simulink model "A_CT_ur10"  (R2021b)
settings: Solver=FixedStepAuto  StartTime=0.0  StopTime=15  FixedStep=1e-3  RelTol=1e1
values from neighbouring files (symbols this model uses):
  Kp = 28*diag([14 14 17 10 22 22])    [GuadagniControllore.m]
  Kv = 32*diag([14 14 17 10 22 22])    [GuadagniControllore.m]
undefined symbols (not defined in the file or in its folder): l1, l2, l3, l4, l5, l6, m1, m2, m3, m4, m5, m6, q0, r
libraries: roblocks x3
(part 1 of 5)
settings Model: Creator=pierg  LastModifiedBy=pierg
settings ModelReferenceCC: ModelReferenceMinAlgLoopOccurrences=on

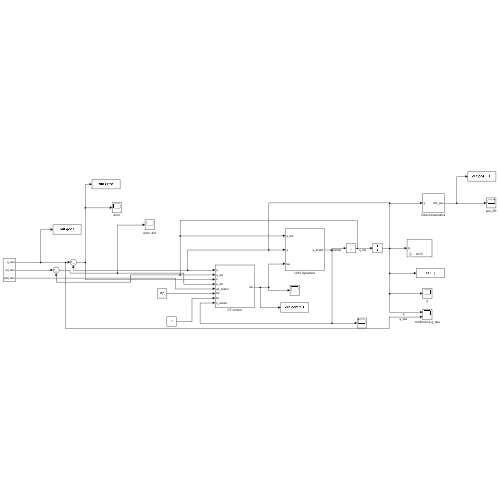
[thumbnail: Simulink's stored preview of the top-level diagram]
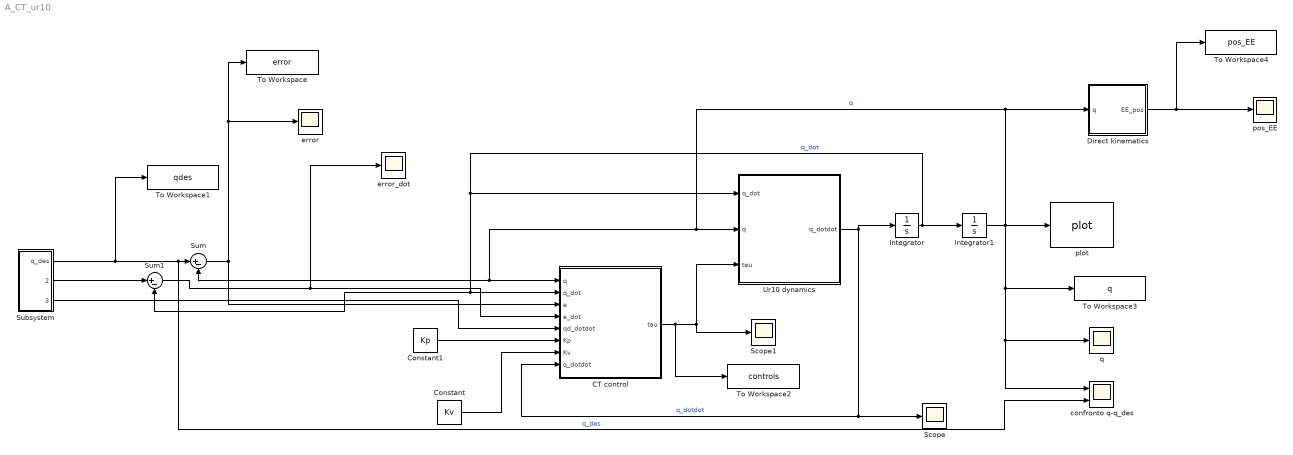
== system A_CT_ur10 ==
  CT control : Subsystem
  Constant : Constant  Value=Kv
  Constant1 : Constant  Value=Kp
  Direct kinematics : Subsystem
  Integrator : Integrator  InitialCondition=[0 0 0 0 0 0]'
  Integrator1 : Integrator  InitialCondition=q0'
  Scope : Scope
  Scope1 : Scope
  Subsystem : Subsystem
  Sum : Sum  Inputs=|+-
  Sum1 : Sum  Inputs=|+-
  To Workspace : ToWorkspace  VariableName=error  SaveFormat=Structure  SampleTime=-1
  To Workspace1 : ToWorkspace  VariableName=qdes  SaveFormat=Structure  SampleTime=-1
  To Workspace2 : ToWorkspace  VariableName=controls  SaveFormat=Structure  SampleTime=-1
  To Workspace3 : ToWorkspace  VariableName=q  SaveFormat=Structure  SampleTime=-1
  To Workspace4 : ToWorkspace  VariableName=pos_EE  SaveFormat=Structure  SampleTime=-1
  Ur10 dynamics : Subsystem
  confronto q-q_des : Scope  NumInputPorts=2
  error : Scope
  error_dot : Scope
  plot : roblocks/Arm/plot  robot=ur10  fps=20  holdplot=on
  pos_EE : Scope
  q : Scope
  wires:
  Ur10 dynamics/1(q_dotdot) -> Integrator/1, CT control/8(q_dotdot), Scope/1  "q_dotdot"
  Integrator/1 -> Integrator1/1, Ur10 dynamics/1(q_dot), Sum1/2, CT control/2(q_dot)  "q_dot"
  Integrator1/1 -> To Workspace3/1, confronto q-q_des/1, q/1, plot/1, Sum/2, CT control/1(q), Ur10 dynamics/2(q), Direct kinematics/1(q)  "q"
  Constant1/1 -> CT control/6(Kp)
  Constant/1 -> CT control/7(Kv)
  Subsystem/1(q_des) -> To Workspace1/1, confronto q-q_des/2, Sum/1  "q_des"
  Subsystem/2(qd_des) -> Sum1/1
  Sum/1 -> CT control/3(e), To Workspace/1, error/1
  Sum1/1 -> error_dot/1, CT control/4(e_dot)
  Subsystem/3(qdd_des) -> CT control/5(qd_dotdot)
  Direct kinematics/1(EE_pos) -> To Workspace4/1, pos_EE/1
  CT control/1(tau) -> To Workspace2/1, Scope1/1, Ur10 dynamics/3(tau)

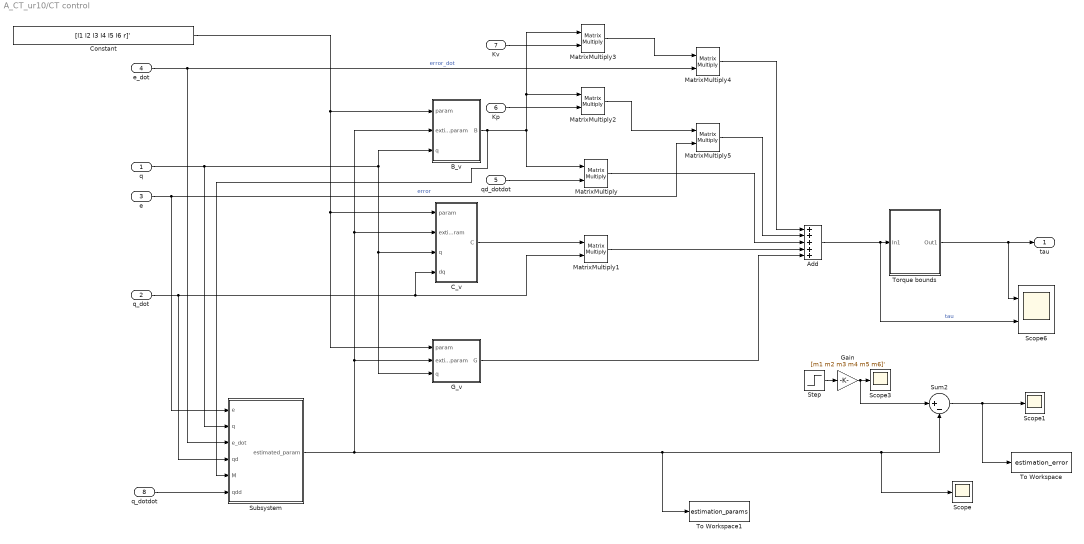
== system A_CT_ur10/CT control ==
  q : Inport
  q_dot : Inport  Port=2
  e : Inport  Port=3
  e_dot : Inport  Port=4
  qd_dotdot : Inport  Port=5
  Kp : Inport  Port=6
  Kv : Inport  Port=7
  q_dotdot : Inport  Port=8
  Add : Sum  Inputs=+++++
  B_v : MATLAB Function  TreatAsAtomicUnit=on
  C_v : MATLAB Function  TreatAsAtomicUnit=on
  Constant : Constant  Value=[l1 l2 l3 l4 l5 l6 r]'
  G_v : MATLAB Function  TreatAsAtomicUnit=on
  Gain : Gain  Gain=[m1 m2 m3 m4 m5 m6]'
  MatrixMultiply{,1..5} (6 alike) : Product  Multiplication=Matrix(*)
  Scope : Scope
  Scope1 : Scope
  Scope3 : Scope
  Scope6 : Scope  NumInputPorts=2
  Step : Step  Before=1  SampleTime=0
  Subsystem : Subsystem
  Sum2 : Sum  Inputs=|+-
  To Workspace : ToWorkspace  VariableName=estimation_error  SaveFormat=Structure  SampleTime=-1
  To Workspace1 : ToWorkspace  VariableName=estimation_params  SaveFormat=Structure  SampleTime=-1
  "Torque bounds " : Subsystem
  tau : Outport
  wires:
  Constant/1 -> G_v/1(param), C_v/1(param), B_v/1(param)
  B_v/1(B) -> Subsystem/5(M), MatrixMultiply/1, MatrixMultiply3/1, MatrixMultiply2/1
  C_v/1(C) -> MatrixMultiply1/1
  q/1 -> Subsystem/2(q), B_v/3(q), G_v/3(q), C_v/3(q)
  q_dot/1 -> Subsystem/4(qd), C_v/4(dq), MatrixMultiply1/2
  Kp/1 -> MatrixMultiply2/2
  Kv/1 -> MatrixMultiply3/2
  e_dot/1 -> Subsystem/3(e_dot), MatrixMultiply4/2  "error_dot"
  MatrixMultiply3/1 -> MatrixMultiply4/1
  MatrixMultiply2/1 -> MatrixMultiply5/1
  e/1 -> Subsystem/1(e), MatrixMultiply5/2  "error"
  MatrixMultiply5/1 -> Add/2
  MatrixMultiply1/1 -> Add/4
  MatrixMultiply4/1 -> Add/1
  MatrixMultiply/1 -> Add/3
  G_v/1(G) -> Add/5
  qd_dotdot/1 -> MatrixMultiply/2
  Sum2/1 -> Scope1/1, To Workspace/1
  Subsystem/1(estimated_param) -> To Workspace1/1, Sum2/2, Scope/1, G_v/2(extimated_param), C_v/2(extimated_param), B_v/2(extimated_param)
  q_dotdot/1 -> Subsystem/6(qdd)
  Step/1 -> Gain/1
  Gain/1 -> Sum2/1, Scope3/1
  Add/1 -> Scope6/2, "Torque bounds "/1(In1)  "tau"
  "Torque bounds "/1(Out1) -> tau/1, Scope6/1

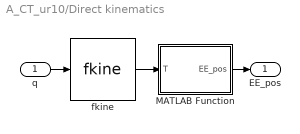
== system A_CT_ur10/Direct kinematics ==
  q : Inport
  MATLAB Function : MATLAB Function  TreatAsAtomicUnit=on
  fkine : roblocks/Arm/fkine  robot=ur10
  EE_pos : Outport
  wires:
  q/1 -> fkine/1
  MATLAB Function/1(EE_pos) -> EE_pos/1
  fkine/1 -> MATLAB Function/1(T)

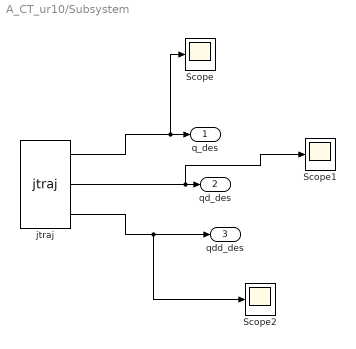
== system A_CT_ur10/Subsystem ==
  Scope : Scope
  Scope1 : Scope
  Scope2 : Scope
  jtraj : roblocks/Toolbox/jtraj  q0=q0  qf=q_des_fin  tmax=15  ts=0.001
  q_des : Outport
  qd_des : Outport  Port=2
  qdd_des : Outport  Port=3
  wires:
  jtraj/1 -> Scope/1, q_des/1
  jtraj/2 -> Scope1/1, qd_des/1
  jtraj/3 -> qdd_des/1, Scope2/1

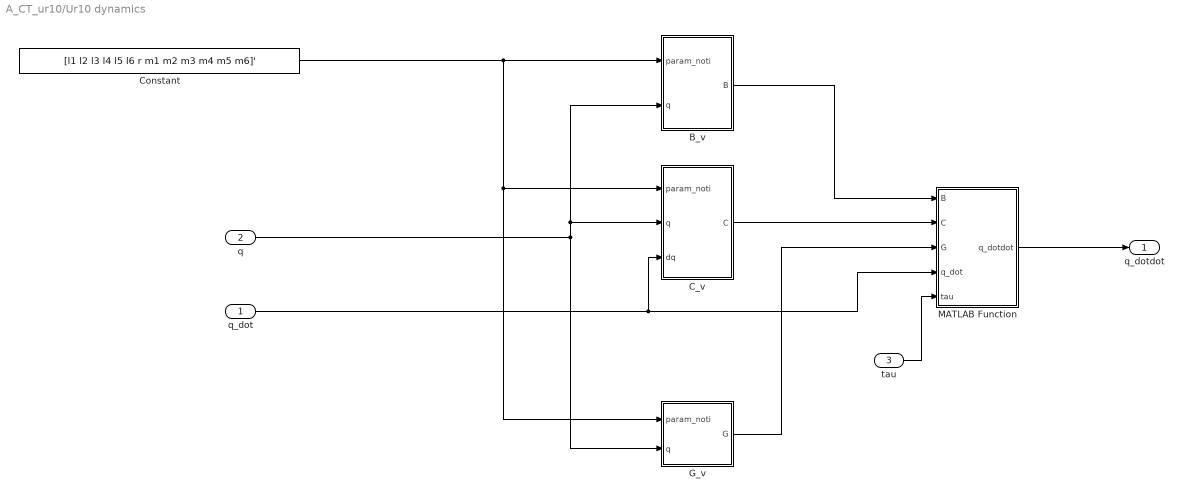
== system A_CT_ur10/Ur10 dynamics ==
  q_dot : Inport
  q : Inport  Port=2
  tau : Inport  Port=3
  B_v : MATLAB Function  TreatAsAtomicUnit=on
  C_v : MATLAB Function  TreatAsAtomicUnit=on
  Constant : Constant  Value=[l1 l2 l3 l4 l5 l6 r m1 m2 m3 m4 m5 m6]'
  G_v : MATLAB Function  TreatAsAtomicUnit=on
  MATLAB Function : MATLAB Function  TreatAsAtomicUnit=on
  q_dotdot : Outport
  wires:
  Constant/1 -> G_v/1(param_noti), C_v/1(param_noti), B_v/1(param_noti)
  q/1 -> B_v/2(q), C_v/2(q), G_v/2(q)
  MATLAB Function/1(q_dotdot) -> q_dotdot/1
  q_dot/1 -> C_v/3(dq), MATLAB Function/4(q_dot)
  tau/1 -> MATLAB Function/5(tau)
  B_v/1(B) -> MATLAB Function/1(B)
  C_v/1(C) -> MATLAB Function/2(C)
  G_v/1(G) -> MATLAB Function/3(G)

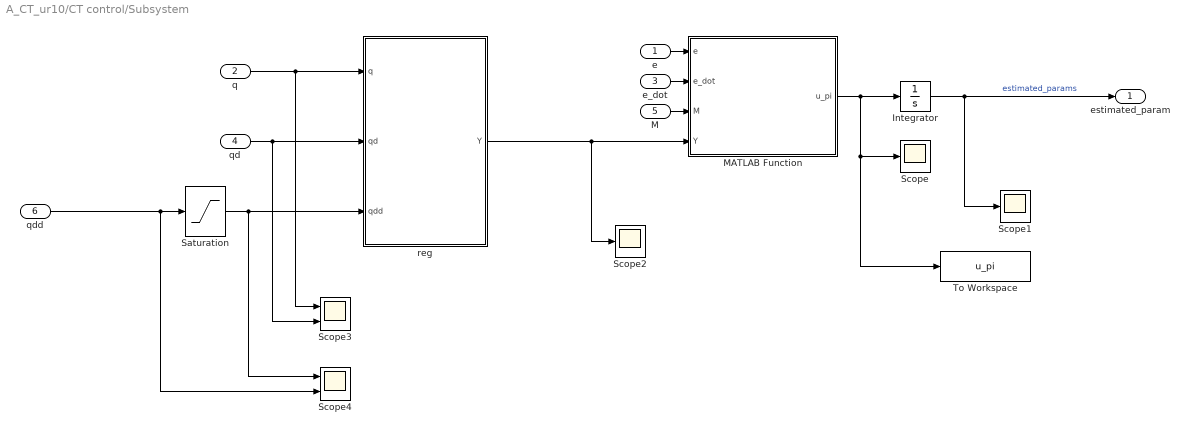
== system A_CT_ur10/CT control/Subsystem ==
  e : Inport
  q : Inport  Port=2
  e_dot : Inport  Port=3
  qd : Inport  Port=4
  M : Inport  Port=5
  qdd : Inport  Port=6
  Integrator : Integrator  InitialCondition=1.2*[m1 m2 m3 m4 m5 m6]'
  MATLAB Function : MATLAB Function  TreatAsAtomicUnit=on
  Saturation : Saturate  UpperLimit=120  LowerLimit=-120
  Scope : Scope
  Scope1 : Scope
  Scope2 : Scope
  Scope3 : Scope  NumInputPorts=2
  Scope4 : Scope  NumInputPorts=2
  To Workspace : ToWorkspace  VariableName=u_pi  SaveFormat=Structure  SampleTime=-1
  reg : MATLAB Function  TreatAsAtomicUnit=on
  estimated_param : Outport
  wires:
  e_dot/1 -> MATLAB Function/2(e_dot)
  Integrator/1 -> Scope1/1, estimated_param/1  "estimated_params"
  e/1 -> MATLAB Function/1(e)
  M/1 -> MATLAB Function/3(M)
  MATLAB Function/1(u_pi) -> To Workspace/1, Scope/1, Integrator/1
  q/1 -> reg/1(q), Scope3/1
  qd/1 -> reg/2(qd), Scope3/2
  qdd/1 -> Scope4/2, Saturation/1
  reg/1(Y) -> Scope2/1, MATLAB Function/4(Y)
  Saturation/1 -> Scope4/1, reg/3(qdd)

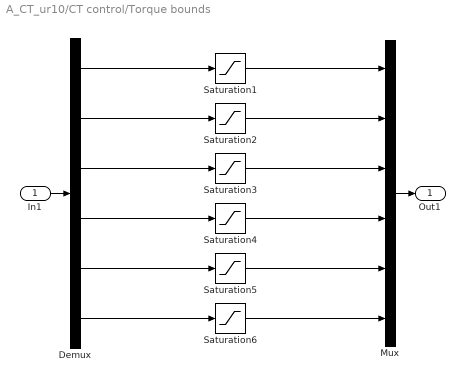
== system A_CT_ur10/CT control/Torque bounds  ==
  In1 : Inport
  Demux : Demux  Outputs=6
  Mux : Mux  Inputs=6
  Saturation1 : Saturate  UpperLimit=330  LowerLimit=-330
  Saturation2 : Saturate  UpperLimit=330  LowerLimit=-330
  Saturation3 : Saturate  UpperLimit=150  LowerLimit=-150
  Saturation4 : Saturate  UpperLimit=56  LowerLimit=-56
  Saturation5 : Saturate  UpperLimit=56  LowerLimit=-56
  Saturation6 : Saturate  UpperLimit=56  LowerLimit=-56
  Out1 : Outport
  wires:
  Demux/3 -> Saturation3/1
  Saturation4/1 -> Mux/4
  Saturation6/1 -> Mux/6
  Saturation1/1 -> Mux/1
  Demux/5 -> Saturation5/1
  Saturation5/1 -> Mux/5
  In1/1 -> Demux/1
  Saturation2/1 -> Mux/2
  Demux/6 -> Saturation6/1
  Demux/4 -> Saturation4/1
  Demux/2 -> Saturation2/1
  Demux/1 -> Saturation1/1
  Saturation3/1 -> Mux/3
  Mux/1 -> Out1/1

== matlab function A_CT_ur10/CT control/Subsystem/MATLAB Function ==
  data: e input; u_pi output; e_dot input; M input; Y input
function u_pi = param_din(e, e_dot, M, Y)
% Definizione matrici della candidata di Lyapunov
R = diag([2 14.8 125 270 275 1490]);
% R(6,6) = 1.0; 
P = 1*eye(12);

% Definizione ingresso di controllo
B = [eye(6); eye(6)];
x = [e; e_dot];
u_pi = R \ (Y' * pinv(M)' * B' * P * x);
